simulink model "Kalman"  (R2021a)
settings: Solver=VariableStepAuto  StartTime=0.0  StopTime=10.0  RelTol=1e-3
undefined symbols (not defined in the file or in its folder): A, Ak, B, b, Bk, C, Ck, Continuous, D, id, iq, K, Kt, Time, w
libraries: ctrlSharedLib x1
settings Model: Creator=migue  LastModifiedBy=migue

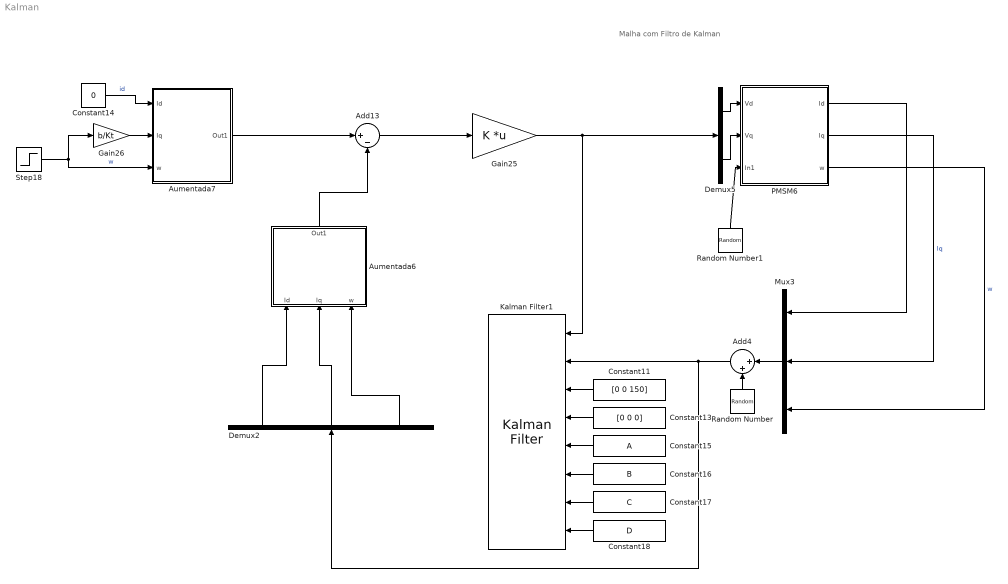
== system Kalman ==
  note: Malha com Filtro de Kalman
  Add13 : Sum  Inputs=|+-
  Add4 : Sum  Inputs=|++
  Aumentada6 : Subsystem
  Aumentada7 : Subsystem
  Constant11 : Constant  Value=[0 0 150]
  Constant13 : Constant  Value=[0 0 0]
  Constant14 : Constant  Value=0
  Constant15 : Constant  Value=A
  Constant16 : Constant  Value=B
  Constant17 : Constant  Value=C
  Constant18 : Constant  Value=D
  Demux2 : Demux  Outputs=3
  Demux5 : Demux  Outputs=2
  Gain25 : Gain  Gain=K  Multiplication=Matrix(K*u)
  Gain26 : Gain  Gain=b/Kt
  Kalman Filter1 : ctrlSharedLib/Kalman Filter  TimeDomain=Continuous-Time  UseCurrentEstimator=on  ModelSource=Input port  ModelSourceVariable=ss(0.95,1,1,0,1)  A=Ak  B=Bk  C=Ck  D=D  NumberOfStates=3  NumberOfInputs=2  NumberOfOutputs=3  InitialEstimateSource=Input port  X0=0  P0=10  UseK=off  UseGH=off  NumberOfProcessNoiseInputs=1  G=1  TimeInvariantG=on  H=0  TimeInvariantH=on  Q=0.05  TimeInvariantQ=on  R=1  TimeInvariantR=on  N=0  TimeInvariantN=on  AddInputPort=on  AddEnablePort=off  OutputEstimatedY=off  OutputP=off  Ts=-1
  Mux3 : Mux  Inputs=3
  PMSM6 : Subsystem  mask{R=0.16, L=1.3e-4, N=10, J=1.8e-4, b=1e-5, lamb=0.06, Kt=0.095}
      mask prompts: R "Resitência (R)"; L "Indutância(L)"; N "Nº de par de polos(N)"; J "coeficiente(J)"; b "coeficiente(b)"; lamb "(lamb)"; Kt "(Kt)"
  Random Number : RandomNumber  SampleTime=0.1
  Random Number1 : RandomNumber  SampleTime=0.1
  Step18 : Step  Before=150  After=151  SampleTime=0
  wires:
  Random Number1/1 -> PMSM6/3(In1)
  Demux5/1 -> PMSM6/1(Vd)
  Demux2/2 -> Aumentada6/2(Iq)
  Gain25/1 -> Demux5/1, Kalman Filter1/1
  Constant16/1 -> Kalman Filter1/6
  Constant15/1 -> Kalman Filter1/5
  Step18/1 -> Aumentada7/3(w), Gain26/1  "w"
  Demux2/3 -> Aumentada6/3(w)
  PMSM6/3(w) -> Mux3/3  "w"
  Mux3/1 -> Add4/1
  Random Number/1 -> Add4/2
  Aumentada6/1(Out1) -> Add13/2
  Add13/1 -> Gain25/1
  Demux5/2 -> PMSM6/2(Vq)
  Constant13/1 -> Kalman Filter1/4
  Constant14/1 -> Aumentada7/1(Id)  "id"
  Constant17/1 -> Kalman Filter1/7
  Aumentada7/1(Out1) -> Add13/1
  Demux2/1 -> Aumentada6/1(Id)
  Constant18/1 -> Kalman Filter1/8
  PMSM6/2(Iq) -> Mux3/2  "Iq"
  Add4/1 -> Demux2/1, Kalman Filter1/2
  PMSM6/1(Id) -> Mux3/1
  Constant11/1 -> Kalman Filter1/3
  Gain26/1 -> Aumentada7/2(Iq)

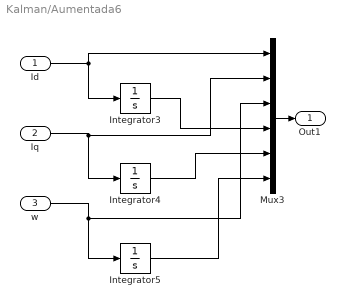
== system Kalman/Aumentada6 ==
  Id : Inport
  Iq : Inport  Port=2
  w : Inport  Port=3
  Integrator3 : Integrator
  Integrator4 : Integrator
  Integrator5 : Integrator
  Mux3 : Mux  Inputs=6
  Out1 : Outport
  wires:
  Iq/1 -> Mux3/2, Integrator4/1
  Id/1 -> Mux3/1, Integrator3/1
  w/1 -> Integrator5/1, Mux3/3
  Integrator3/1 -> Mux3/4
  Integrator5/1 -> Mux3/6
  Mux3/1 -> Out1/1
  Integrator4/1 -> Mux3/5

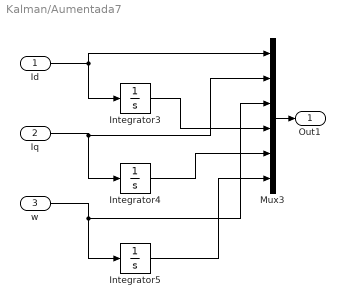
== system Kalman/Aumentada7 ==
  Id : Inport
  Iq : Inport  Port=2
  w : Inport  Port=3
  Integrator3 : Integrator
  Integrator4 : Integrator
  Integrator5 : Integrator
  Mux3 : Mux  Inputs=6
  Out1 : Outport
  wires:
  Iq/1 -> Mux3/2, Integrator4/1
  Id/1 -> Mux3/1, Integrator3/1
  w/1 -> Integrator5/1, Mux3/3
  Integrator3/1 -> Mux3/4
  Integrator5/1 -> Mux3/6
  Mux3/1 -> Out1/1
  Integrator4/1 -> Mux3/5

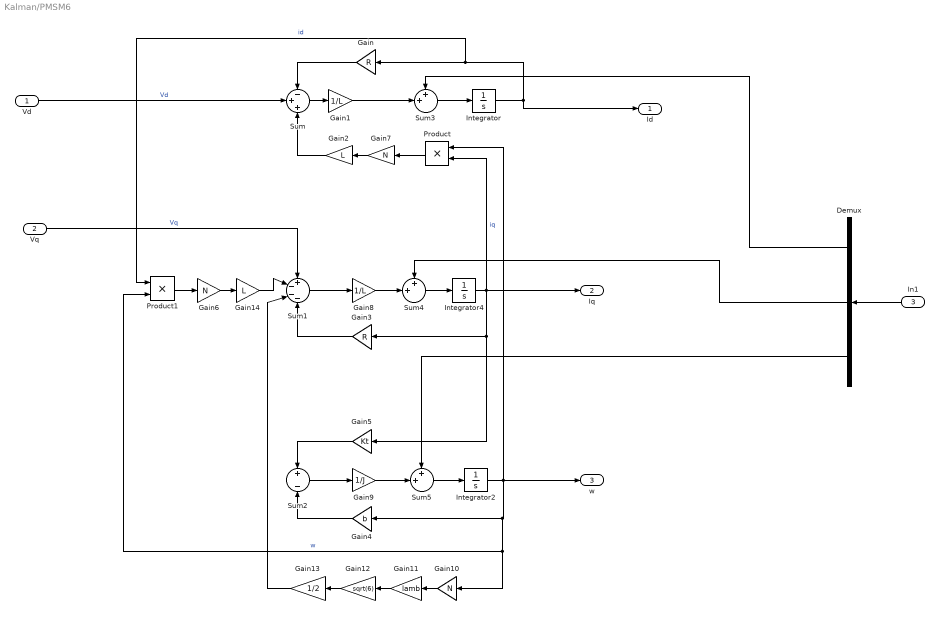
== system Kalman/PMSM6 ==
  Vd : Inport
  Vq : Inport  Port=2
  In1 : Inport  Port=3
  Demux : Demux  Outputs=3
  Gain : Gain  Gain=R
  Gain1 : Gain  Gain=1/L
  Gain10 : Gain  Gain=N
  Gain11 : Gain  Gain=lamb
  Gain12 : Gain  Gain=sqrt(6)
  Gain13 : Gain  Gain=1/2
  Gain14 : Gain  Gain=L
  Gain2 : Gain  Gain=L
  Gain3 : Gain  Gain=R
  Gain4 : Gain  Gain=b
  Gain5 : Gain  Gain=Kt
  Gain6 : Gain  Gain=N
  Gain7 : Gain  Gain=N
  Gain8 : Gain  Gain=1/L
  Gain9 : Gain  Gain=1/J
  Integrator : Integrator  InitialCondition=id
  Integrator2 : Integrator  InitialCondition=w
  Integrator4 : Integrator  InitialCondition=iq
  Product : Product
  Product1 : Product
  Sum : Sum  Inputs=-++
  Sum1 : Sum  Inputs=+---
  Sum2 : Sum  Inputs=+-
  Sum3 : Sum  Inputs=++|
  Sum4 : Sum  Inputs=++|
  Sum5 : Sum  Inputs=++|
  Id : Outport
  Iq : Outport  Port=2
  w : Outport  Port=3
  wires:
  Integrator4/1 -> Iq/1, Product/2, Gain3/1, Gain5/1  "iq"
  Integrator/1 -> Gain/1, Product1/1, Id/1  "id"
  Sum1/1 -> Gain8/1
  Product1/1 -> Gain6/1
  Gain/1 -> Sum/1
  Sum2/1 -> Gain9/1
  Integrator2/1 -> w/1, Product/1, Gain10/1, Product1/2, Gain4/1  "w"
  Gain5/1 -> Sum2/1
  Vd/1 -> Sum/2  "Vd"
  Sum/1 -> Gain1/1
  Gain4/1 -> Sum2/2
  Gain3/1 -> Sum1/4
  Gain11/1 -> Gain12/1
  Gain10/1 -> Gain11/1
  Product/1 -> Gain7/1
  Vq/1 -> Sum1/1  "Vq"
  Gain12/1 -> Gain13/1
  Gain13/1 -> Sum1/3
  Gain6/1 -> Gain14/1
  Gain7/1 -> Gain2/1
  Gain2/1 -> Sum/3
  Gain14/1 -> Sum1/2
  Gain1/1 -> Sum3/2
  Sum3/1 -> Integrator/1
  Sum4/1 -> Integrator4/1
  Gain8/1 -> Sum4/2
  Sum5/1 -> Integrator2/1
  Gain9/1 -> Sum5/2
  Demux/1 -> Sum3/1
  Demux/2 -> Sum4/1
  Demux/3 -> Sum5/1
  In1/1 -> Demux/1
